simulink model "plane"  (R2015b)
settings: Solver=FixedStepAuto  StartTime=0.0  StopTime=t_sim  FixedStep=0.02  RelTol=1e-3
values from neighbouring files (symbols this model uses):
  omega_alpha = []    [State.m]    (also in Vehicle.m = movementCommand(1))
  omega_beta = []    [State.m]    (also in Vehicle.m = movementCommand(2))
  omega_gamma = []    [State.m]    (also in Vehicle.m = movementCommand(3))
  velocity = []    [State.m]    (also in Vehicle.m = movementCommand(4))
undefined symbols (not defined in the file or in its folder): omega_alpha_0, omega_beta_0, omega_gamma_0, x_0, y_0, z_0
settings Model: Creator=H172461  LastModifiedBy=H172461

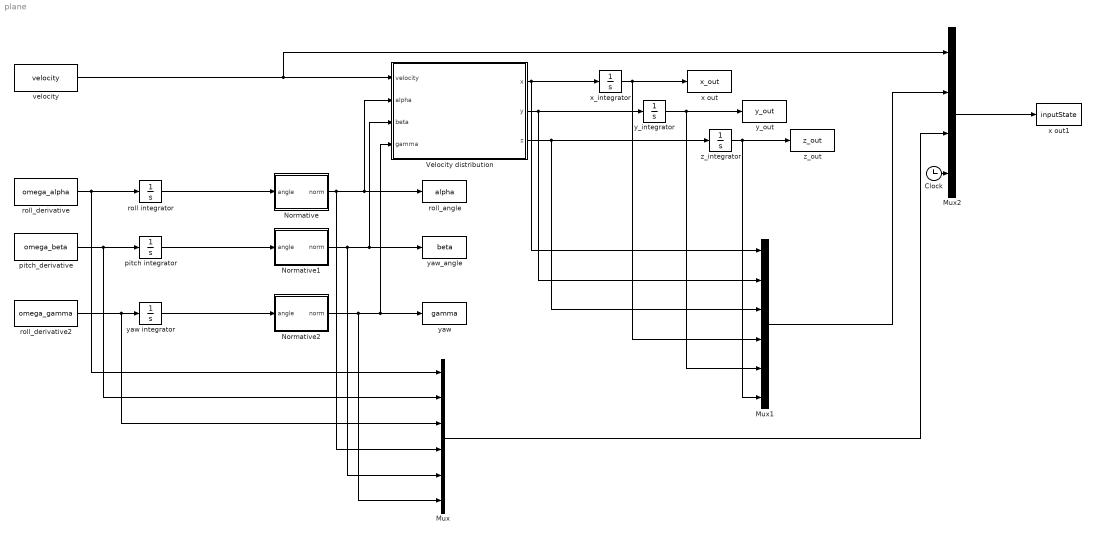
== system plane ==
  Clock : Clock
  Mux : Mux  Inputs=6
  Mux1 : Mux  Inputs=6
  Mux2 : Mux
  Normative : MATLAB Function  TreatAsAtomicUnit=on
  Normative1 : MATLAB Function  TreatAsAtomicUnit=on
  Normative2 : MATLAB Function  TreatAsAtomicUnit=on
  Velocity distribution : MATLAB Function  TreatAsAtomicUnit=on
  pitch integrator : Integrator  InitialCondition=omega_beta_0
  pitch_derivative : Constant  Value=omega_beta
  roll integrator : Integrator  InitialCondition=omega_alpha_0
  roll_angle : ToWorkspace  VariableName=alpha  SampleTime=-1
  roll_derivative : Constant  Value=omega_alpha
  roll_derivative2 : Constant  Value=omega_gamma
  velocity : Constant  Value=velocity
  x out : ToWorkspace  VariableName=x_out  SampleTime=-1
  x out1 : ToWorkspace  VariableName=inputState  SampleTime=-1
  x_integrator : Integrator  InitialCondition=x_0
  y_integrator : Integrator  InitialCondition=y_0
  y_out : ToWorkspace  VariableName=y_out  SampleTime=-1
  yaw : ToWorkspace  VariableName=gamma  SampleTime=-1
  yaw integrator : Integrator  InitialCondition=omega_gamma_0
  yaw_angle : ToWorkspace  VariableName=beta  SampleTime=-1
  z_integrator : Integrator  InitialCondition=z_0
  z_out : ToWorkspace  VariableName=z_out  SampleTime=-1
  wires:
  roll_derivative/1 -> roll integrator/1, Mux/1
  roll integrator/1 -> Normative/1(angle)
  Normative/1(norm) -> Mux/4, Velocity distribution/2(alpha), roll_angle/1
  pitch_derivative/1 -> pitch integrator/1, Mux/2
  pitch integrator/1 -> Normative1/1(angle)
  Normative1/1(norm) -> Mux/5, Velocity distribution/3(beta), yaw_angle/1
  roll_derivative2/1 -> Mux/3, yaw integrator/1
  yaw integrator/1 -> Normative2/1(angle)
  Normative2/1(norm) -> Mux/6, Velocity distribution/4(gamma), yaw/1
  velocity/1 -> Mux2/1, Velocity distribution/1(velocity)
  Velocity distribution/1(x) -> x_integrator/1, Mux1/1
  Velocity distribution/2(y) -> Mux1/2, y_integrator/1
  Velocity distribution/3(z) -> Mux1/3, z_integrator/1
  x_integrator/1 -> x out/1, Mux1/4
  y_integrator/1 -> Mux1/5, y_out/1
  z_integrator/1 -> Mux1/6, z_out/1
  Mux1/1 -> Mux2/2
  Mux/1 -> Mux2/3
  Clock/1 -> Mux2/4
  Mux2/1 -> x out1/1

== matlab function plane/Normative1 ==
  data: angle input; norm output
function norm = fcn(angle)
%#codegen
norm = atan2(sin(angle),cos(angle));

== matlab function plane/Normative ==
  data: angle input; norm output
function norm = fcn(angle)
%#codegen
norm = atan2(sin(angle),cos(angle));

== matlab function plane/Normative2 ==
  data: angle input; norm output
function norm = fcn(angle)
%#codegen
norm = atan2(sin(angle),cos(angle));

== matlab function plane/Velocity distribution ==
  data: x output; velocity input; y output; alpha input; beta input; gamma input; z output
function [x,y,z] = fcn(velocity, alpha,beta, gamma)
%#codegen
v= [velocity;0;0];
ROT = [ cos(beta)*cos(gamma), cos(gamma)*sin(alpha)*sin(beta) - cos(alpha)*sin(gamma), sin(alpha)*sin(gamma) + cos(alpha)*cos(gamma)*sin(beta);
 cos(beta)*sin(gamma), cos(alpha)*cos(gamma) + sin(alpha)*sin(beta)*sin(gamma), cos(alpha)*sin(beta)*sin(gamma) - cos(gamma)*sin(alpha);
           -sin(beta),                                    cos(beta)*sin(alpha),                                    cos(alpha)*cos(beta)];
 v_dist=ROT*v;
 
 x=v_dist(1);
 y=v_dist(2);
 z=v_dist(3);
